simulink model "DC_motor"  (R2022b)
settings: Solver=FixedStepAuto  StartTime=0.0  StopTime=inf  RelTol=1e-3  EnableMultiTasking=on
libraries: arduinolib x9, Arduino_Additional_Lib x1, arduinosensorlib x1
settings Model: ExtModeTrigDuration=2  Creator=hyundaiAuto  LastModifiedBy=hyundaiAuto
settings OptimizationCC: EnhancedBackFolding=on  PassReuseOutputArgsAs=Individual arguments  ZeroExternalMemoryAtStartup=off  ZeroInternalMemoryAtStartup=off  MaxStackSize=64  OptimizeBlockOrder=speed  DifferentSizesBufferReuse=on  OptimizationCustomize=off  EfficientTunableParamExpr=on
settings DebuggingCC: MultiTaskRateTransMsg=warning  ParameterTunabilityLossMsg=error
settings HardwareCC: ProdBitPerInt=16  ProdBitPerPointer=16  ProdBitPerSizeT=16  ProdBitPerPtrDiffT=16  ProdLargestAtomicFloat=None  ProdWordSize=8  ProdHWDeviceType=Atmel->AVR
settings SFSimCC: MATLABDynamicMemAlloc=off
settings RTWCC: Description=Embedded Coder  SystemTargetFile=ert.tlc  HardwareBoard=Arduino Mega 2560  TLCOptions=-aInlineSetEventsForThisBaseRateFcn=TLC_FALSE -aSuppressMultiTaskScheduler=TLC_FALSE -aRateBasedStepFcn=1  TemplateMakefile=ert_default_tmf  Toolchain=Arduino AVR  BuildConfiguration=Faster Runs
settings CodeAppCC: ForceParamTrailComments=on  IgnoreCustomStorageClasses=off  OperatorAnnotations=on  SimulinkDataObjDesc=on  SFDataObjDesc=on  InsertBlockDesc=on
settings ERTTargetCC: SupportContinuousTime=on  SupportVariableSizeSignals=on  ExtModeTransport=3  ExtModeStaticAlloc=on  ExtModeAutomaticAllocSize=off  ExtModeStaticAllocSize=2048  ExtModeMexFile=ext_xcp  ExtModeIntrfLevel=Level2 - Open

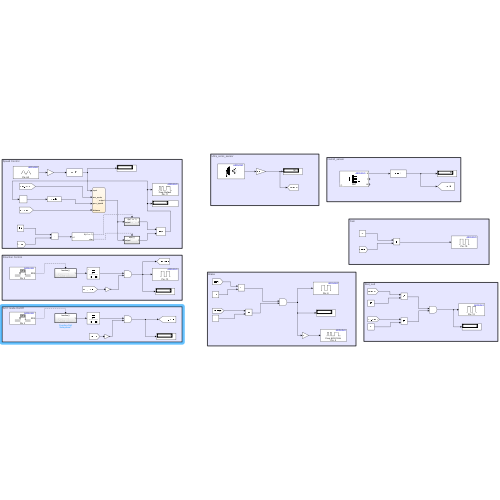
[thumbnail: Simulink's stored preview of the top-level diagram]
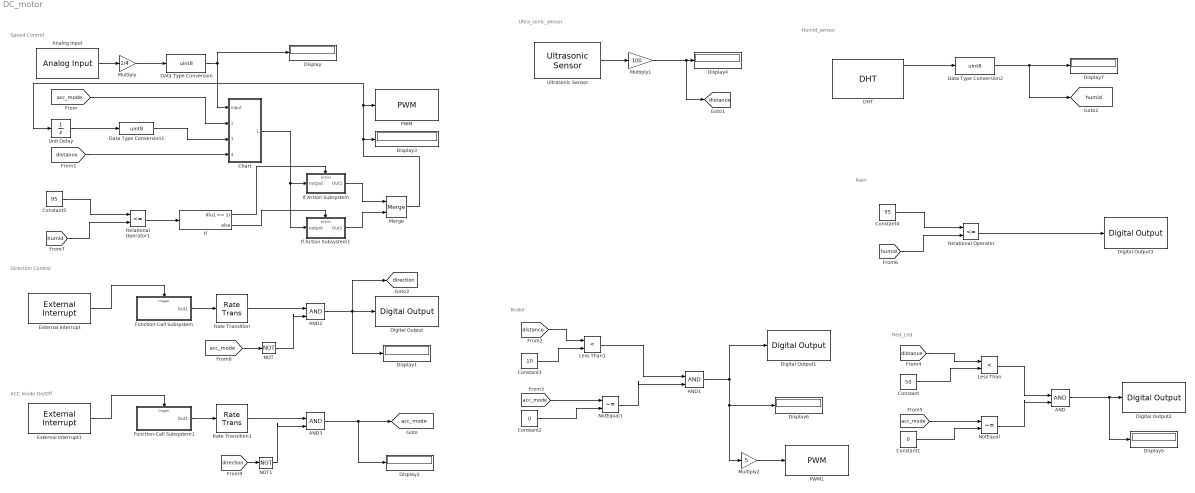
== system DC_motor ==
  note: Rain
  note: Humid_sensor
  note: Brake
  note: Speed Control
  note: Direction Control
  note: ACC mode On/Off
  note: Ultra_sonic_sensor
  note: Red_Led
  AND{,1..3} (4 alike) : Logic  IconShape=distinctive  AllPortsSameDT=off  OutDataTypeStr=boolean
  Analog Input : arduinolib/Analog Input  pinNumber=0  ReadResultsOnly=off  ConversionTriggerSource=Software  ExternalTriggerType=uint32( 0 )  OutputDataType=uint16  EnableConversionCompleteNotify=off  EnableOuputStatus=off  SampleTime=-1  blockPlatform=arduino
  Chart : Stateflow chart  TreatAsAtomicUnit=on
      settings: PortSchema="{\"entries\":[{\"content\":{\"sides\":[{\"content\":{\"connectorIds\":[\"In2\",\"In1\",\"In3\",\"In4\"]},\"type\":\"ConnectorPlacement.EquallySpacedRectSide\",\"uuid\":\"d0de167e-cbb5-436d-a976-1cd6a91270d1\"},{\"content\":{\"connectorIds\":[\"Out1\"],\"side\":\"RIGHT\"},\"type\":\"ConnectorPlacement.EquallySpacedRectSide\",\"uuid\":\"99f56787-17d8-459e-a573-14fd5ee0d26a\"},{\"content\":{\"connectorIds\":[],\"side\":\"TOP\"},\"type\":\"ConnectorPlacement.EquallySpacedRectSide\",\"uuid\":\"d5f56c18-0116-4037-a466-3def5a444482\"}]},\"type\":\"ConnectorPlacement.EquallySpacedConnector\",\"uuid\":\"e3f14907-94e9-49f6-a412-5fdfc9c57e34\"}],\"packageUris\":[\"http://schema.mathworks.com/mf0/Connector/R2020b\"],\"version\":\"1.0\"}"
  Constant : Constant  Value=50
  Constant1 : Constant  Value=0
  Constant2 : Constant  Value=0
  Constant3 : Constant  Value=10
  Constant4 : Constant  Value=95
  Constant5 : Constant  Value=95
  DHT : Arduino_Additional_Lib/DHT  F=off  Pin=4  Tp=11  Ts=0.5
      settings: SourceProductName=Arduino Additional Sensors Library
  Data Type Conversion : DataTypeConversion  OutDataTypeStr=uint8  SaturateOnIntegerOverflow=off  RndMeth=Floor
  Data Type Conversion1 : DataTypeConversion  OutDataTypeStr=uint8  SaturateOnIntegerOverflow=off  RndMeth=Floor
  Data Type Conversion2 : DataTypeConversion  OutDataTypeStr=uint8  SaturateOnIntegerOverflow=off  RndMeth=Floor
  Digital Output : arduinolib/Digital Output  pinNumber=13  Direction=output  blockPlatform=arduino
  Digital Output1 : arduinolib/Digital Output  pinNumber=8  Direction=output  blockPlatform=arduino
  Digital Output2 : arduinolib/Digital Output  pinNumber=12  Direction=output  blockPlatform=arduino
  Digital Output3 : arduinolib/Digital Output  pinNumber=10  Direction=output  blockPlatform=arduino
  Display{,1..7} (8 alike) : Display
  External Interrupt : arduinolib/External Interrupt  Pin=2  PullUp=off  Mode=FALLING  InterruptSimulationInput=off
  External Interrupt1 : arduinolib/External Interrupt  Pin=3  PullUp=off  Mode=FALLING  InterruptSimulationInput=off
  Function-Call Subsystem : Subsystem  TreatAsAtomicUnit=on
  Function-Call Subsystem1 : Subsystem  TreatAsAtomicUnit=on
  If : If  IfExpression=u1 == 1
  If Action Subsystem : Subsystem  TreatAsAtomicUnit=on
  If Action Subsystem1 : Subsystem  TreatAsAtomicUnit=on
  Less Than : RelationalOperator  Operator=<  OutDataTypeStr=boolean  RndMeth=Simplest  InputSameDT=off
  Less Than1 : RelationalOperator  Operator=<  OutDataTypeStr=boolean  RndMeth=Simplest  InputSameDT=off
  Merge : Merge
  Multiply : Gain  Gain=1/4
  Multiply1 : Gain  Gain=100
  Multiply2 : Gain  Gain=5
  NOT : Logic  Operator=NOT  IconShape=distinctive  AllPortsSameDT=off  OutDataTypeStr=boolean
  NOT1 : Logic  Operator=NOT  IconShape=distinctive  AllPortsSameDT=off  OutDataTypeStr=boolean
  NotEqual : RelationalOperator  Operator=~=  OutDataTypeStr=boolean  RndMeth=Simplest  InputSameDT=off
  NotEqual1 : RelationalOperator  Operator=~=  OutDataTypeStr=boolean  RndMeth=Simplest  InputSameDT=off
  PWM : arduinolib/PWM  pinNumber=11  frequencyType=Default  desiredFrequency=490.2  achievableFrequency=490.2
  PWM1 : arduinolib/PWM  pinNumber=5  frequencyType=Specify  desiredFrequency=622.25  achievableFrequency=622.2291
  Rate Transition : RateTransition  Deterministic=off
  Rate Transition1 : RateTransition  Deterministic=off
  Relational Operator : RelationalOperator  Operator=<=  OutDataTypeStr=boolean  RndMeth=Simplest  InputSameDT=off
  Relational Operator1 : RelationalOperator  Operator=<=  OutDataTypeStr=boolean  RndMeth=Simplest  InputSameDT=off
  Ultrasonic Sensor : arduinosensorlib/Ultrasonic Sensor  NumSignalPins=2  TrigPin=50  EchoPin=51  SignalPin=3  SampleTime_=0.1  blockPlatform=ARDUINO
  Unit Delay : UnitDelay  SampleTime=-1  HasFrameUpgradeWarning=on
  tag scope: acc_mode=global, direction=global, distance=global, humid=global
  wires:
  Data Type Conversion/1 -> Chart/2(input), Display/1
  Analog Input/1 -> Multiply/1
  Multiply/1 -> Data Type Conversion/1
  Function-Call Subsystem/1(Out1) -> Rate Transition/1
  External Interrupt/1 -> Function-Call Subsystem/Trigger
  Chart/1(output) -> If Action Subsystem1/1(output), If Action Subsystem/1(output)
  [acc_mode] -> Chart/1(acc_mode)
  External Interrupt1/1 -> Function-Call Subsystem1/Trigger
  Function-Call Subsystem1/1(Out1) -> Rate Transition1/1
  Unit Delay/1 -> Data Type Conversion1/1
  Data Type Conversion1/1 -> Chart/3(prev_speed)
  Ultrasonic Sensor/1 -> Multiply1/1
  Multiply1/1 -> [distance], Display4/1
  [distance] -> Chart/4(distance)
  [distance] -> Less Than/1
  Constant/1 -> Less Than/2
  [acc_mode] -> NotEqual/1
  Constant1/1 -> NotEqual/2
  Less Than/1 -> AND/1
  NotEqual/1 -> AND/2
  AND/1 -> Display5/1, Digital Output2/1
  [distance] -> Less Than1/1
  Constant3/1 -> Less Than1/2
  Constant2/1 -> NotEqual1/2
  [acc_mode] -> NotEqual1/1
  Less Than1/1 -> AND1/1
  NotEqual1/1 -> AND1/2
  AND1/1 -> Multiply2/1, Display6/1, Digital Output1/1
  Multiply2/1 -> PWM1/1
  DHT/1 -> Data Type Conversion2/1
  Data Type Conversion2/1 -> [humid], Display7/1
  [humid] -> Relational Operator/2
  Constant4/1 -> Relational Operator/1
  Relational Operator/1 -> Digital Output3/1
  [humid] -> Relational Operator1/2
  Constant5/1 -> Relational Operator1/1
  Relational Operator1/1 -> If/1
  If/1 -> If Action Subsystem/Action
  If/2 -> If Action Subsystem1/Action
  If Action Subsystem1/1(Out1) -> Merge/2
  If Action Subsystem/1(Out1) -> Merge/1
  Merge/1 -> Unit Delay/1, PWM/1, Display3/1
  Rate Transition/1 -> AND2/1
  [acc_mode] -> NOT/1
  NOT/1 -> AND2/2
  AND2/1 -> [direction], Digital Output/1, Display1/1
  AND3/1 -> Display2/1, [acc_mode]
  Rate Transition1/1 -> AND3/1
  [direction] -> NOT1/1
  NOT1/1 -> AND3/2

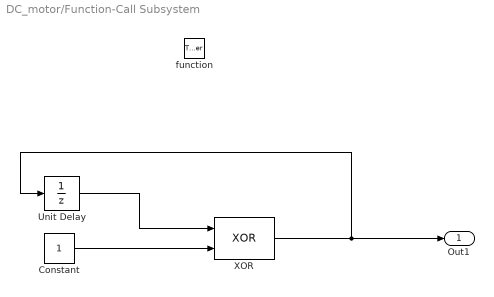
== system DC_motor/Function-Call Subsystem ==
  function : TriggerPort  TriggerType=function-call  VariantControl=(inherit)
  Constant : Constant
  Unit Delay : UnitDelay  SampleTime=-1  HasFrameUpgradeWarning=on
  XOR : Logic  Operator=XOR  IconShape=distinctive  AllPortsSameDT=off  OutDataTypeStr=boolean
  Out1 : Outport
  wires:
  Constant/1 -> XOR/2
  Unit Delay/1 -> XOR/1
  XOR/1 -> Unit Delay/1, Out1/1

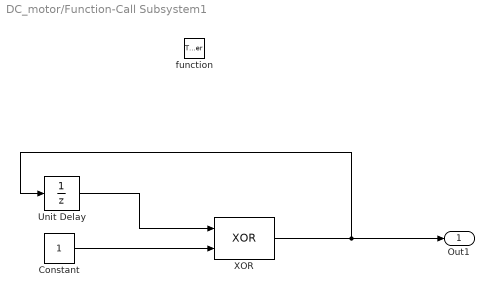
== system DC_motor/Function-Call Subsystem1 ==
  function : TriggerPort  TriggerType=function-call  VariantControl=(inherit)
  Constant : Constant
  Unit Delay : UnitDelay  SampleTime=-1  HasFrameUpgradeWarning=on
  XOR : Logic  Operator=XOR  IconShape=distinctive  AllPortsSameDT=off  OutDataTypeStr=boolean
  Out1 : Outport  OutDataTypeStr=boolean
  wires:
  Constant/1 -> XOR/2
  Unit Delay/1 -> XOR/1
  XOR/1 -> Unit Delay/1, Out1/1

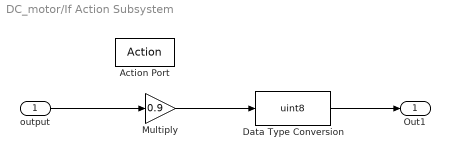
== system DC_motor/If Action Subsystem ==
  output : Inport
  Action Port : ActionPort  ActionPortLabel=if(u1 == 1)
  Data Type Conversion : DataTypeConversion  OutDataTypeStr=uint8  SaturateOnIntegerOverflow=off  RndMeth=Floor
  Multiply : Gain  Gain=0.9
  Out1 : Outport
  wires:
  output/1 -> Multiply/1
  Multiply/1 -> Data Type Conversion/1
  Data Type Conversion/1 -> Out1/1

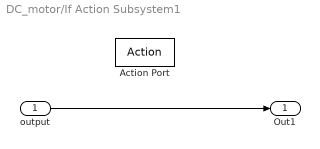
== system DC_motor/If Action Subsystem1 ==
  output : Inport
  Action Port : ActionPort  ActionPortLabel=else
  Out1 : Outport
  wires:
  output/1 -> Out1/1

== stateflow chart DC_motor/Chart ==
  state acc_off
    output = input;
    acc_speed = prev_speed
  state speed_control
    output = acc_speed;
  state return
    acc_speed = 60;
  state follow
    output = acc_speed * 0.9;
  state follow_4
    output = 0;
  state follow_1
    output = acc_speed * 0.8;
  state follow_2
    output = acc_speed * 0.7;
  state follow_3
    output = acc_speed * 0.6;
  (default) -> acc_off
  acc_off -> speed_control : [acc_mode > 0]
  return -> speed_control
  speed_control -> acc_off [order 1] : [acc_mode == 0]
  speed_control -> follow [order 2] : [distance <= 50]
  follow -> speed_control [order 3] : [acc_speed > 60 && distance > 50]
  follow -> return [order 1] : [acc_speed < 60 && distance > 50]
  follow -> follow_1 [order 2] : [distance <=40 && distance > 30]
  follow_1 -> follow [order 2] : [distance > 40]
  follow_3 -> follow_4 [order 2] : [distance < 10]
  follow_4 -> follow_3 : [distance >= 10]
  follow_1 -> follow_2 [order 1] : [distance <= 30 && distance > 20]
  follow_2 -> follow_1 [order 2] : [distance > 30]
  follow_2 -> follow_3 [order 1] : [distance <= 20 && distance >= 10]
  follow_3 -> follow_2 [order 1] : [distance > 20]
  data: acc_mode input; output output; input input; prev_speed input; distance input; acc_speed local
